simulink subsystem "BEV4EMSSC"  (R2024a)
settings: Solver=VariableStepAuto  StartTime=0.0  StopTime=10.0  RelTol=1e-3
undefined symbols (not defined in the file): DriveshftTrq1, DriveshftTrq2, DriveshftTrq3, DriveshftTrq4, EM1, EM2, EM3, EM4
libraries: fl_lib x4
settings Model: ModifiedByFormat=The MathWorks, Inc.  Creator=The MathWorks, Inc.  LastModifiedBy=The MathWorks, Inc.
settings OptimizationCC: ReuseModelBlockBuffer=off
settings DebuggingCC: SubsystemReferenceDiagnosticForUnitTest=warning
settings RTWCC: GPUComputeCapability=3.5

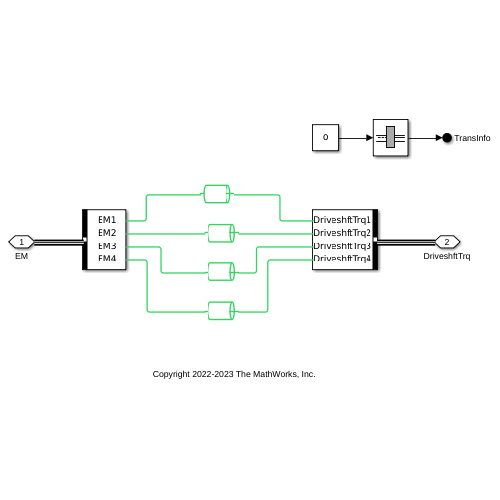
[thumbnail: Simulink's stored preview of the top-level diagram]
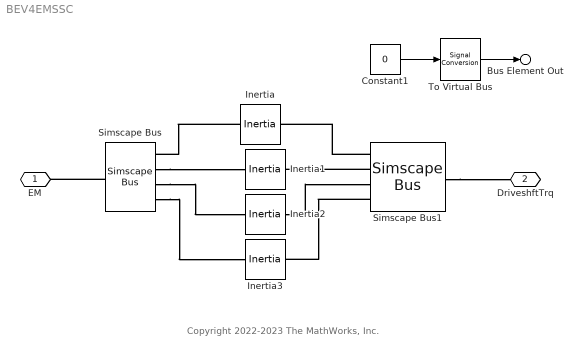
== system BEV4EMSSC ==
  note: Copyright 2022-2023 The MathWorks, Inc.
  Constant1 : Constant  Value=0  OutDataTypeStr=Bus: TransInfoBUS  SampleTime=Inf
  Inertia : fl_lib/Mechanical/Rotational Elements/Inertia  inertia=PlntEM1RotInertia kg*m^2  num_ports=foundation.enum.numPorts2.two  w_specify=off  w_priority=High  w=0 rad/s  w_nominal_specify=off  w_nominal_value=1  w_nominal_unit=rad/s  t_specify=off  t_priority=None  t=0 N*m  t_nominal_specify=off  t_nominal_value=1  t_nominal_unit=N*m
      settings: InternalSimscapePortConfiguration="{\"Bottom\":[],\"Left\":[{\"id\":\"I\",\"label\":\"\",\"type\":\"foundation.mechanical.rotational.rotational\"}],\"Right\":[{\"id\":\"J\",\"label\":\"\",\"type\":\"foundation.mechanical.rotational.rotational\"}],\"Top\":[]}"
  Inertia1 : fl_lib/Mechanical/Rotational Elements/Inertia  inertia=PlntEM2RotInertia kg*m^2  num_ports=foundation.enum.numPorts2.two  w_specify=off  w_priority=High  w=0 rad/s  w_nominal_specify=off  w_nominal_value=1  w_nominal_unit=rad/s  t_specify=off  t_priority=None  t=0 N*m  t_nominal_specify=off  t_nominal_value=1  t_nominal_unit=N*m
      settings: InternalSimscapePortConfiguration="{\"Bottom\":[],\"Left\":[{\"id\":\"I\",\"label\":\"\",\"type\":\"foundation.mechanical.rotational.rotational\"}],\"Right\":[{\"id\":\"J\",\"label\":\"\",\"type\":\"foundation.mechanical.rotational.rotational\"}],\"Top\":[]}"
  Inertia2 : fl_lib/Mechanical/Rotational Elements/Inertia  inertia=PlntEM3RotInertia kg*m^2  num_ports=foundation.enum.numPorts2.two  w_specify=off  w_priority=High  w=0 rad/s  w_nominal_specify=off  w_nominal_value=1  w_nominal_unit=rad/s  t_specify=off  t_priority=None  t=0 N*m  t_nominal_specify=off  t_nominal_value=1  t_nominal_unit=N*m
      settings: InternalSimscapePortConfiguration="{\"Bottom\":[],\"Left\":[{\"id\":\"I\",\"label\":\"\",\"type\":\"foundation.mechanical.rotational.rotational\"}],\"Right\":[{\"id\":\"J\",\"label\":\"\",\"type\":\"foundation.mechanical.rotational.rotational\"}],\"Top\":[]}"
  Inertia3 : fl_lib/Mechanical/Rotational Elements/Inertia  inertia=PlntEM4RotInertia kg*m^2  num_ports=foundation.enum.numPorts2.two  w_specify=off  w_priority=High  w=0 rad/s  w_nominal_specify=off  w_nominal_value=1  w_nominal_unit=rad/s  t_specify=off  t_priority=None  t=0 N*m  t_nominal_specify=off  t_nominal_value=1  t_nominal_unit=N*m
      settings: InternalSimscapePortConfiguration="{\"Bottom\":[],\"Left\":[{\"id\":\"I\",\"label\":\"\",\"type\":\"foundation.mechanical.rotational.rotational\"}],\"Right\":[{\"id\":\"J\",\"label\":\"\",\"type\":\"foundation.mechanical.rotational.rotational\"}],\"Top\":[]}"
  Simscape Bus : SimscapeBus  HierarchyStrings=EM1;EM2;EM3;EM4
  Simscape Bus1 : SimscapeBus  HierarchyStrings=DriveshftTrq1;DriveshftTrq2;DriveshftTrq3;DriveshftTrq4
  To Virtual Bus : SignalConversion  ConversionOutput=Virtual bus  OverrideOpt=off
  EM : PMIOPort  Side=Left
  DriveshftTrq : PMIOPort  Port=2  Side=Right
  Bus Element Out : Outport  PortName=TransInfo
  wires:
  Constant1/1 -> To Virtual Bus/1
  To Virtual Bus/1 -> Bus Element Out/1
  connections:
  Inertia/RConn1 -- Simscape Bus/LConn1
  Simscape Bus/LConn2 -- Inertia1/RConn1
  Simscape Bus/LConn3 -- Inertia2/RConn1
  Simscape Bus/LConn4 -- Inertia3/RConn1
  Simscape Bus/RConn1 -- EM/RConn1
  Simscape Bus1/RConn1 -- DriveshftTrq/RConn1
  Simscape Bus1/LConn1 -- Inertia/LConn1
  Simscape Bus1/LConn2 -- Inertia1/LConn1
  Inertia2/LConn1 -- Simscape Bus1/LConn3
  Simscape Bus1/LConn4 -- Inertia3/LConn1
